simulink model "cast_surge"  (R2018b)
settings: Solver=FixedStepAuto  StartTime=0.0  StopTime=50  FixedStep=0.1  RelTol=1e-3
libraries: simulink x1
settings Model: Creator=Kellan  LastModifiedBy=Kellan

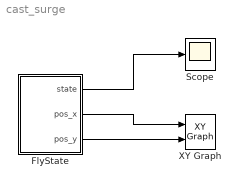
== system cast_surge ==
  FlyState : Stateflow chart  TreatAsAtomicUnit=on
  Scope : Scope
  XY Graph : simulink/Sinks/XY Graph  xmin=-10  xmax=210  ymin=-10  ymax=210  st=-1
  wires:
  FlyState/1(state) -> Scope/1
  FlyState/2(pos_x) -> XY Graph/1
  FlyState/3(pos_y) -> XY Graph/2

== stateflow chart cast_surge/FlyState ==
  state Initialize
    en:
    pos_x = 50
    pos_y = 0
    upwind = [0.1; 1]
    upwind = upwind/norm(upwind)
  state Cast
    en:
    state=1;
    state Leftward
      en:
      th = pi/2
      dir = [cos(th),-sin(th);sin(th),cos(th)]*upwind
      dir = dir + normrnd(0,0.1, 2, 1)
      du:
      pos_x = pos_x + dir(1)
      pos_y = pos_y + dir(2)
      check_target(pos_x, pos_y)
      check_scent(pos_x, pos_y)
    state Rightward
      en:
      th = -pi/2
      dir = [cos(th),-sin(th);sin(th),cos(th)]*upwind
      normrnd(0,0.1, 2, 1)
      du:
      pos_x = pos_x + dir(1)
      pos_y = pos_y + dir(2)
      check_target(pos_x, pos_y)
      check_scent(pos_x, pos_y)
    (default) -> (junction 39)
    (junction 39) -> Rightward [order 1] : [rand>0.5]
    (junction 39) -> Leftward [order 2]
    Leftward -> Rightward : [rand>0.9]
    Rightward -> Leftward : [rand>0.9]
  state Done
    en:
    state=4
  state Surge
    en:
    state=2
    du:
    dir = upwind + normrnd(0,0.1, 2, 1)
    pos_x = pos_x + dir(1)
    pos_y = pos_y + dir(2)
    check_target(pos_x, pos_y)
    check_scent(pos_x, pos_y)
  (default) -> Initialize
  Initialize -> Cast
  Cast -> Done [order 1] : TARGET_REACHED
  Cast -> Surge [order 2] : SCENT_TRUE
  Surge -> Cast [order 2] : SCENT_FALSE
  Surge -> Done [order 1] : TARGET_REACHED
  data: x function_input; y function_input; x function_input; y function_input; state output; pos_x output; pos_y output; th local; upwind local; dir local
  events: SCENT_FALSE local FUNCTION_CALL_EVENT; SCENT_TRUE local FUNCTION_CALL_EVENT; TARGET_REACHED local FUNCTION_CALL_EVENT
  function check_scent(x,y):
    | function check_scent(x,y)
    | 
    | gauss = @(x,x0,s)exp(-(x-x0).^2/(2*s^2));
    | if rand < gauss(x, 100, 10)*0.9
    |     send(SCENT_TRUE)
    | else
    |     send(SCENT_FALSE)
    | end
  function check_target(x,y):
    | function check_target(x,y)
    |  
    | target = [100; 200];
    | if norm([x;y] - target) < 10
    |     send(TARGET_REACHED)
    | end
